simulink model "log_data"  (R2017b)
settings: Solver=FixedStepDiscrete  StartTime=0.0  StopTime=10.0  RelTol=1e-3
undefined symbols (not defined in the file or in its folder): RGBLED_COLOR_ENUM, RGBLED_MODE_ENUM
libraries: pixhawk_slib_sensors_actuators x4
settings Model: Creator=wsh  LastModifiedBy=Mr Wang
settings OptimizationCC: DefaultParameterBehavior=Inlined  MaxStackSize=64
settings DebuggingCC: ParameterTunabilityLossMsg=error
settings HardwareCC: ProdBitPerPointer=32  ProdBitPerSizeT=32  ProdBitPerPtrDiffT=32  ProdLargestAtomicInteger=Long  ProdLargestAtomicFloat=Double  ProdWordSize=32  ProdHWDeviceType=ARM Compatible->ARM Cortex
settings SFSimCC: MATLABDynamicMemAlloc=off
settings RTWCC: SystemTargetFile=ert.tlc  HardwareBoard=Pixhawk PX4  TemplateMakefile=ert_default_tmf  GenerateReport=on  Toolchain=Pixhawk Toolchain  IncludeHyperlinkInReport=on  LaunchReport=on  GenerateTraceInfo=on  GenerateTraceReport=on  GenerateTraceReportSl=on  GenerateTraceReportSf=on  GenerateTraceReportEml=on
settings CodeAppCC: ForceParamTrailComments=on  IgnoreCustomStorageClasses=off  OperatorAnnotations=on  SimulinkDataObjDesc=on  SFDataObjDesc=on  MATLABFcnDesc=on  InsertBlockDesc=on  StateflowObjectComments=on  MATLABSourceComments=on
settings ERTTargetCC: MultiwordLength=2048  ERTCustomFileTemplate=PX4_codertarget_file_process.tlc

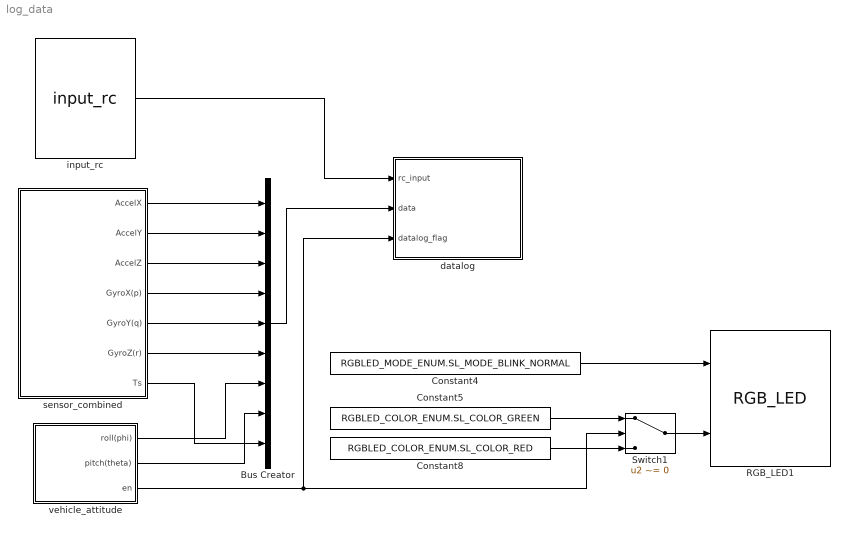
== system log_data ==
  Bus Creator : BusCreator  Inputs=9
  Constant4 : Constant  Value=RGBLED_MODE_ENUM.SL_MODE_BLINK_NORMAL  OutDataTypeStr=Enum: RGBLED_MODE_ENUM
  Constant5 : Constant  Value=RGBLED_COLOR_ENUM.SL_COLOR_GREEN  OutDataTypeStr=Enum: RGBLED_COLOR_ENUM
  Constant8 : Constant  Value=RGBLED_COLOR_ENUM.SL_COLOR_RED  OutDataTypeStr=Enum: RGBLED_COLOR_ENUM
  RGB_LED1 : pixhawk_slib_sensors_actuators/RGB_LED  Description=|
      | This block gives the user control over various lighting modes of the RGB LED available on the PX4 hardware. 
      | This block accepts 2 inputs: Mode and Color.  These are enumeration data types.  You can find out what values are valid in the MATLAB command window by typing: 
      | Enumeration members for class 'RGBLED_COLOR_ENUM':
      |     SL_COLOR_OFF
      |     SL_COLOR_RED
      |     SL_COLOR_GREEN
      |     SL_COLOR_BLUE
      |     SL_COLOR_YELLOW
      |     SL_COLOR_PURPLE
      |     SL_COLOR_AMBER
      |     SL_COLOR_CYAN
      |     SL_COLOR_WHITE 
      | Enumeration members for class 'RGBLED_MODE_ENUM':
      |     SL_MODE_OFF
      |     SL_MODE_ON
      |     SL_MODE_DISABLED
      |     SL_MODE_BLINK_SLOW
      |     SL_MODE_BLINK_NORMAL
      |     SL_MODE_BLINK_FAST
      |     SL_MODE_BREATHE  
      | Look at the sample Simulink model: px4demo_rgbled.slx for an example of how to use this block.
      settings: SourceProductName=Pixhawk Target Blocks
  Switch1 : Switch  Criteria=u2 ~= 0  Threshold=1500
  "datalog " : Subsystem
  input_rc : pixhawk_slib_sensors_actuators/input_rc  Description=|  sampletime=1/250  channel1=off  channel2=off  channel3=off  channel4=off  channel5=on  channel6=off  channel7=off  channel8=off  channel9=off  channel10=off  channel11=off  channel12=off  channel13=off  channel14=off  channel15=off  channel16=off  channel17=off  channel18=off  ch_count=off  rssi=off  rc_failsafe=off  rc_lost=off  rc_inputsource=off
      | RC Input Block
      | 
      | This block provides user input control to the model.
      | It uses the input_rc uORB topic.
      | 
      | The user has the ability to choose which channels are available as outputs from this block and also some optional outputs. These include 
      | Channels 1 through 18
      | double data type indicating the PWM value from the controller 
      | measured pulse widths for each of the supported channels 
      | Channel Count 
      | uint32 data type of the number of channels which are detector by the PX4 
      | RC Failsafe 
      | boolean data types indicating that the RC Tx is sending the FailSafe signal (if equipped and properly setup) 
      | explicit failsafe flag: true on TX failure or TX out of range , false otherwise. 
      | Only the true state is reliable, as there are some (PPM) receivers on the market going into failsafe without telling us explicitly. 
      | RC Input Source 
      | Enumeration data type indicating which source the RC input is from. 
      | Valid values are found in the ENUM file: RC_INPUT_SOURCE_ENUM.m 
      |           Enumeration members for class 'RC_INPUT_SOURCE_ENUM':
      |           RCINPUT_SOURCE_UNKNOWN         (0)
      |           RCINPUT_SOURCE_PX4FMU_PPM      (1)
      |           RCINPUT_SOURCE_PX4IO_PPM       (2)
      |           RCINPUT_SOURCE_PX4IO_SPEKTRUM  (3)
      |           RCINPUT_SOURCE_PX4IO_SBUS      (4)
      |           RCINPUT_SOURCE_PX4IO_ST24      (5)
      |           RCINPUT_SOURCE_MAVLINK         (6)
      |           RCINPUT_SOURCE_QURT            (7)
      |           RCINPUT_SOURCE_PX4FMU_SPEKTRUM (8)
      |           RCINPUT_SOURCE_PX4FMU_SBUS     (9)
      |           RCINPUT_SOURCE_PX4FMU_ST24     (10)
      |           RCINPUT_SOURCE_PX4FMU_SUMD     (11)
      |           RCINPUT_SOURCE_PX4FMU_DSM      (12)
      |           RCINPUT_SOURCE_PX4IO_SUMD      (13)
      | 
      | RSSI - Receive signal strength index 
      | receive signal strength indicator (RSSI): < 0: Undefined, 0: no signal, 255: full reception 
      | RC Lost Connection 
      | boolean data type indicating RC receiver connection status 
      | True, if no frame has arrived in the expected time, false otherwise. 
      | True usally means that the receiver has been disconnected, but can also indicate a radio link loss on "stupid" systems. 
      | Will remain false, if a RX with failsafe option continues to transmit frames after a link loss. 
      |   
      | Sample Model: px4demo_input_rc.slx
      settings: SourceProductName=Pixhawk Target Blocks
  "sensor_combined   " : Subsystem
  "vehicle_attitude    " : Subsystem
  wires:
  Bus Creator/1 -> "datalog "/2(data)
  "sensor_combined   "/1(AccelX) -> Bus Creator/1
  "sensor_combined   "/2(AccelY) -> Bus Creator/2
  "sensor_combined   "/3(AccelZ) -> Bus Creator/3
  "sensor_combined   "/4(GyroX(p)) -> Bus Creator/4
  "sensor_combined   "/5(GyroY(q)) -> Bus Creator/5
  "sensor_combined   "/6(GyroZ(r)) -> Bus Creator/6
  "vehicle_attitude    "/1(roll(phi)) -> Bus Creator/7
  "vehicle_attitude    "/2(pitch(theta)) -> Bus Creator/8
  input_rc/1 -> "datalog "/1(rc_input)
  "sensor_combined   "/7(Ts) -> Bus Creator/9
  "vehicle_attitude    "/3(en) -> Switch1/2, "datalog "/3(datalog_flag)
  Constant8/1 -> Switch1/3
  Constant5/1 -> Switch1/1
  Switch1/1 -> RGB_LED1/2
  Constant4/1 -> RGB_LED1/1

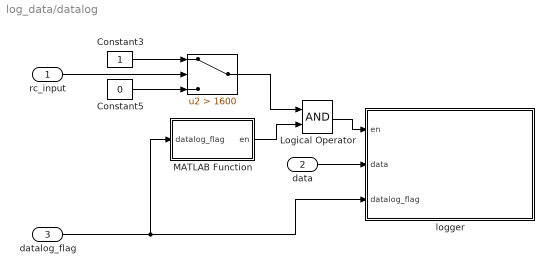
== system log_data/datalog  ==
  rc_input : Inport
  data : Inport  Port=2
  datalog_flag : Inport  Port=3
  " " : Switch  Criteria=u2 > Threshold  Threshold=1600
  Constant3 : Constant
  Constant5 : Constant  Value=0
  Logical Operator : Logic  AllPortsSameDT=off  OutDataTypeStr=boolean
  MATLAB Function : MATLAB Function  TreatAsAtomicUnit=on
  logger : Subsystem  mask(Binary Logger){logfile=/fs/microsd/log/e4, cacheflag=off, numRecs=60000}
      mask prompts: cacheflag "Cache in Memory"; numRecs "Max Record Count"
      mask help:
      | Log a vector of data to a file on the SD card
      |
      | If Cache in Memory is on data is written when en goes low or when max number of records specified is reached.
      | Otherwise Max Number of Records is used to indicate when to performa an fflush out to file.
      mask init:
      | logname=uint8(logfile);
      mask Help: eval('pixhawk.internal.doc(''binary_logger_Block.html'')');
      mask Display:
      | fprintf(get_param(gcb,'logfile'))
      | port_label('input',1,'en')
      | port_label('input',2,'data')
      | port_label('input',3,'datalog_flag')
  wires:
  rc_input/1 -> " "/2
  data/1 -> logger/2(data)
  datalog_flag/1 -> logger/3(datalog_flag), MATLAB Function/1(datalog_flag)
  Constant3/1 -> " "/1
  Constant5/1 -> " "/3
  " "/1 -> Logical Operator/1
  MATLAB Function/1(en) -> Logical Operator/2
  Logical Operator/1 -> logger/1(en)

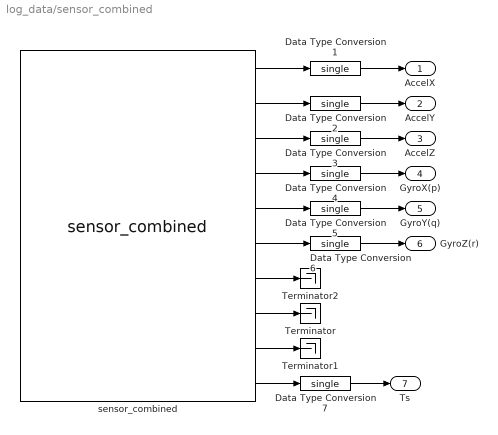
== system log_data/sensor_combined    ==
  Data Type Conversion{1..7} (7 alike) : DataTypeConversion  OutDataTypeStr=single
  Terminator : Terminator
  Terminator1 : Terminator
  Terminator2 : Terminator
  sensor_combined : pixhawk_slib_sensors_actuators/sensor_combined  Description=|  sampletime=1/250  show_mag=off  show_acc=on  show_gyro=on  show_baro=off  show_ts=on
      | Sensor Combined Block
      | 
      | This block enables access to the various sensors available on the px4fmu-v2 hardware.  
      | The user can use these signals in the Simulink control model.  
      | The sample time needs to be provided in the mask dialog.  
      | Optional output ports can also be selected.  
      | Refer to the sample model: px4demo_attitude_control.slx
      | 
      | Signal definitions: 
      | Magnetometer (x,y,z) - single values – Magnetic field in NED body frame, in Gauss 
      | Accelerometer (x,y,z) - single values – Acceleration in NED body frame, in m/s^2 
      | Gyroscope (p,q,r) - single values – Angular velocity in radians per second 
      | Barometer (Altitude) - single value – Barometric pressure, already temperature compensated (millibars) 
      | RunTime (timestamp) - double value – Timestamp in microseconds since boot, from gyro 
      |   
      | The sensor_combined block needs to have the px4io service running on the PX4 hardware in order to get valid signal values.
      settings: SourceProductName=Pixhawk Target Blocks
  AccelX : Outport
  AccelY : Outport  Port=2
  AccelZ : Outport  Port=3
  GyroX(p) : Outport  Port=4
  GyroY(q) : Outport  Port=5
  GyroZ(r) : Outport  Port=6
  Ts : Outport  Port=7
  wires:
  sensor_combined/7 -> Terminator2/1
  Data Type Conversion1/1 -> AccelX/1
  Data Type Conversion4/1 -> GyroX(p)/1
  sensor_combined/5 -> Data Type Conversion5/1
  Data Type Conversion3/1 -> AccelZ/1
  Data Type Conversion5/1 -> GyroY(q)/1
  sensor_combined/4 -> Data Type Conversion4/1
  Data Type Conversion2/1 -> AccelY/1
  Data Type Conversion7/1 -> Ts/1
  Data Type Conversion6/1 -> GyroZ(r)/1
  sensor_combined/1 -> Data Type Conversion1/1
  sensor_combined/2 -> Data Type Conversion2/1
  sensor_combined/3 -> Data Type Conversion3/1
  sensor_combined/6 -> Data Type Conversion6/1
  sensor_combined/9 -> Terminator1/1
  sensor_combined/8 -> Terminator/1
  sensor_combined/10 -> Data Type Conversion7/1

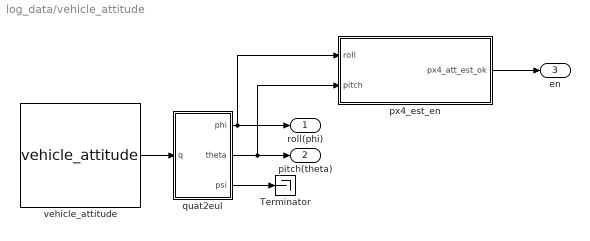
== system log_data/vehicle_attitude     ==
  Terminator : Terminator
  px4_est_en : MATLAB Function  TreatAsAtomicUnit=on
  quat2eul : MATLAB Function  TreatAsAtomicUnit=on
  vehicle_attitude : pixhawk_slib_sensors_actuators/vehicle_attitude  Description=|  sampletime=0.004  show_r=off  show_p=off  show_y=off  show_q=on  show_ts=off
      | This block gives access to the running service that calculates the vehicle’s attitude.  A uORB topic (vehicle_attitude (attitude measurements)) publisher MUST be running in order for this block to provide valid signal values.  The available ones as of v1.3 are: 
      | attitude_estimator_ekf – EKF-Extended Kalman Filter for attitude estimation 
      | attitude_estimator_so3 – SO(3)-attitude estimation by using accelerometer, gyroscopes and magnetometer 
      | One of these MUST be running on the px4fmu in order for this block to return valid values.  Refer to the sample model: px4demo_attitude_control.slx. Attitude in NED (North-East-Down) body frame in SI units. 
      | Signal definitions: 
      | Roll – single value, Roll angle (rad, Tait-Bryan, NED) 
      | Pitch – single value, Pitch angle (rad, Tait-Bryan, NED) 
      | Yaw – single value, Yaw angle (rad, Tait-Bryan, NED) 
      | Quaternion (NED) – single(4) values (optional based on the uORB publisher)
      settings: SourceProductName=Pixhawk Target Blocks
  roll(phi) : Outport
  pitch(theta) : Outport  Port=2
  en : Outport  Port=3
  wires:
  quat2eul/1(phi) -> px4_est_en/1(roll), roll(phi)/1
  quat2eul/2(theta) -> px4_est_en/2(pitch), pitch(theta)/1
  quat2eul/3(psi) -> Terminator/1
  vehicle_attitude/1 -> quat2eul/1(q)
  px4_est_en/1(px4_att_est_ok) -> en/1

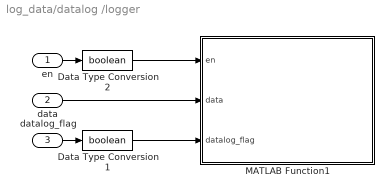
== system log_data/datalog /logger ==
  en : Inport
  data : Inport  Port=2
  datalog_flag : Inport  Port=3
  Data Type Conversion1 : DataTypeConversion  OutDataTypeStr=boolean
  Data Type Conversion2 : DataTypeConversion  OutDataTypeStr=boolean
  MATLAB Function1 : MATLAB Function  TreatAsAtomicUnit=on
  wires:
  data/1 -> MATLAB Function1/2(data)
  Data Type Conversion2/1 -> MATLAB Function1/1(en)
  en/1 -> Data Type Conversion2/1
  datalog_flag/1 -> Data Type Conversion1/1
  Data Type Conversion1/1 -> MATLAB Function1/3(datalog_flag)

== matlab function log_data/datalog /logger/MATLAB Function1 ==
  data: en input boolean; data input; datalog_flag input boolean; logname parameter uint8; cacheflag parameter boolean; numRecs parameter uint32
%% Binary Logger
% Note: All data needs to be of the same type (e.g. double)
% Header information format:
%           String "MWLOGV##"
%           Time/Date 4 bytes (time())
%           Number of Signals per record Logged 1 byte (256 max)
%           Data Type of Signals Logged  1 byte (1-10)
%           Number of bytes per record 2 bytes (65535 max)
% This does NOT include the number of data sets logged.  
% i.e. The Reader is responsible for reading until EOF.
% MathWorks Pilot Engineering 2015
% Steve Kuznicki
function binary_logger(en, data, datalog_flag, logname, cacheflag, numRecs)
%#codegen
    persistent fp isflushed isopen count lognumstr elem_size vect_size
    coder.cinclude('<stdio.h>');
    coder.cinclude('<time.h>');
    
    if isempty(count)
        count = uint32(0);
        lognumstr = 65;
        isopen = false;
        fp = coder.opaque('FILE*', 'NULL');
        isflushed = false;
        elem_size = uint16(1);
        vect_size = coder.const(uint8(numel(data)));
        if cacheflag == true
            %datastored = zeros(numRecs*uint32(coder.const(numel(data))), 1, 'like', data);
        end
    end

    if (en)
        if isopen == false
            [elsize, eltype] = get_elem_size(data);
            elem_size = coder.const(uint16(elsize));
            elem_type = coder.const(uint8(eltype));
            vect_size = coder.const(uint8(numel(data)));
            coder.ceval('printf',['OPENING file %s vect_size %d elem_size %d numRecs %d %c' uint8(0)], ...
                [logname, '_', char(lognumstr), '.bin', int8(0)], uint32(vect_size), uint32(elem_size), uint32(numRecs), uint8(10));
            fp = coder.ceval('fopen', [logname, '_', char(lognumstr), '.bin', int8(0)], ['wb', int8(0)]);
            lognumstr = lognumstr + 1;
            isflushed = false;
            count = uint32(0);
            isopen = true;
            % Write header information here
            % header token + version
            mlStrVer = 'MWLOGV01';
            coder.ceval('fwrite', coder.rref(mlStrVer), uint32(1), length(mlStrVer), fp);
            % date/time
            tm = uint32(0);
            tmptr = uint32(0);
            tm = coder.ceval('time',coder.wref(tmptr));
            coder.ceval('fwrite', coder.rref(tm), uint32(4), uint32(1), fp);
            % number of elements in each record
            coder.ceval('fwrite', coder.rref(vect_size), uint32(1), uint32(1), fp);
            % data type of the elements
            coder.ceval('fwrite', coder.rref(elem_type), uint32(1), uint32(1), fp);
            % size of each record in bytes
            recSize = elem_size * uint16(vect_size);
            coder.ceval('fwrite', coder.rref(recSize), uint32(2), uint32(1), fp);
        end
        % cache data in memory or use fwrite
        if cacheflag == true
            addr = (count*uint32(vect_size))+1;
            for idx = 1:vect_size
                %datastored(addr) = data(idx);
                addr = addr + 1;
            end
            count = count + uint32(1);
        else
            if  datalog_flag
                coder.ceval('fwrite', coder.rref(data), elem_size, vect_size, fp);
                count = count + uint32(1);
            end
        end
        
        % check for data count limit
        if count >= numRecs
            if cacheflag
                for idx = 1:count*uint32(vect_size)
                    %coder.ceval('fwrite', coder.rref(datastored(idx)), elem_size, uint32(1), fp);
                end
            end
            coder.ceval('fflush', fp);
            isflushed = false;
            count = uint32(0);
        end
    else
        if isopen == true
            if ~isflushed 
                coder.ceval('printf',['CLOSING file. count = %d %c' uint8(0)], uint32(count), uint8(10));
                if cacheflag
                    count = count + uint32(1);
                    for idx = 1:count*uint32(vect_size)
                        %coder.ceval('fwrite', coder.rref(datastored(idx)), elem_size, uint32(1), fp);
                    end
                end
                coder.ceval('fflush', fp);
                isflushed = true;
            end
            coder.ceval('fclose', fp);
        end
        isopen = false;
        count = uint32(0);
    end
end

% return the size of the element in bytes
function [elem_size, dtype] = get_elem_size(data)
    switch(class(data))
        case 'double'
            elem_size = 8;
            dtype = 1;
        case 'single'
            elem_size = 4;
            dtype = 2;
        case 'int32'
            elem_size = 4;
            dtype = 3;
        case 'uint32'
            elem_size = 4;
            dtype = 4;
        case 'int16'
            elem_size = 2;
            dtype = 5;
        case 'uint16'
            elem_size = 2;
            dtype = 6;
        case 'int8'
            elem_size = 1;
            dtype = 7;
        case 'uint8'
            elem_size = 1;
            dtype = 8;
        case 'logical'
            elem_size = 1;
            dtype = 9;
        case 'embedded.fi'
            nt = numerictype(data);
            elem_size = 2^ceil(log2(ceil(nt.WordLength / 8)));
            dtype = 10;
    end
    if ~isreal(data)
        elem_size = elem_size*2;
    end
    
    elem_size = uint16(elem_size);
    dtype = uint8(dtype);
end

== matlab function log_data/vehicle_attitude    /px4_est_en ==
  data: roll input; px4_att_est_ok output; pitch input
function px4_att_est_ok = px4_est_en(roll, pitch)

if abs(roll) < 0.000001 && abs(pitch) < 0.000001
    px4_att_est_ok = false;
else
    px4_att_est_ok = true;
end

== matlab function log_data/datalog /MATLAB Function ==
  data: datalog_flag input; en output
function en = fcn(datalog_flag)

persistent count;
if isempty(count)
    count = 0;
end

if datalog_flag
    count = count + 1;
end
if count > 60000
    en = false;
    count = 0;
else
    en = true;
end

== matlab function log_data/vehicle_attitude    /quat2eul ==
  data: q input; phi output; theta output; psi output
function [phi,theta,psi] = quat2eul(q)
% Conversion from Quaternion to Euler angles based on the PX4 Firmware
% v1.6.5 release.
% 
% Quaternion -> DCM -> Euler Angles
% INPUT:
%   q: Quaternion vector of the format: (a + bi + cj + dk)
% OUTPUT:
%   [phi,theta,psi]: Euler angles in radians.
% 
 
    a = q(1);
    b = q(2);
    c = q(3);
    d = q(4);

    aSq = a*a;
    bSq = b*b;
    cSq = c*c;
    dSq = d*d;

    d_pi2 = pi/2;

    % quaternion_to_dcm
    dcm00 = aSq + bSq - cSq - dSq;
    % dcm01 = 2*(b*c - a*d);
    dcm02 = 2*(a*c + b*d);
    dcm10 = 2*(b*c + a*d);
    % dcm11 = aSq - bSq + cSq - dSq;
    dcm12 = 2*(c*d - a*b);
    dcm20 = 2*(b*d - a*c);
    dcm21 = 2*(a*b + c*d);
    dcm22 = aSq - bSq - cSq + dSq;

    % dcm_to_euler
    theta = asin(-dcm20);
    if abs(theta - d_pi2) < 1.0e-3
        phi = single(0.0);
        psi = atan2(dcm12, dcm02);
    elseif abs(theta + d_pi2) < 1.0e-3
        phi = single(0.0);
        psi = atan2(-dcm12, -dcm02);
    else
        phi = atan2(dcm21, dcm22);
        psi = atan2(dcm10, dcm00);
    end

end
